simulink model "schem_3_2"  (R2024a)
settings: Solver=VariableStepAuto  StartTime=0.0  StopTime=25  RelTol=1e-3
undefined symbols (not defined in the file): G11, G12, G21, G22, G23, xi_120, xi_220, xi_230
settings Model: Creator=user  LastModifiedBy=user

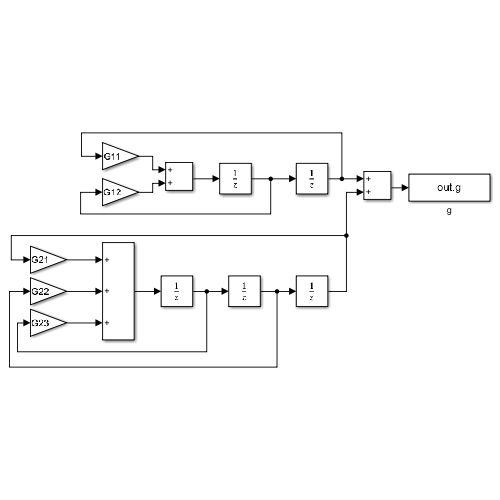
[thumbnail: Simulink's stored preview of the top-level diagram]
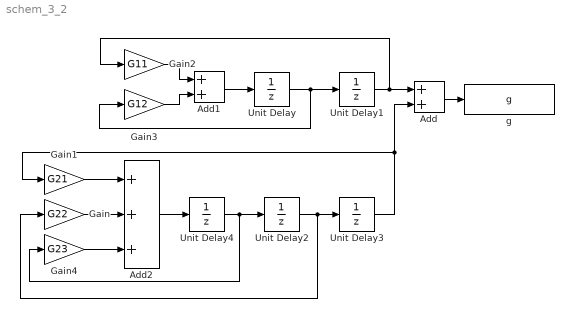
== system schem_3_2 ==
  Add : Sum
  Add1 : Sum
  Add2 : Sum  Inputs=+++
  Gain : Gain  Gain=G22
  Gain1 : Gain  Gain=G21
  Gain2 : Gain  Gain=G11
  Gain3 : Gain  Gain=G12
  Gain4 : Gain  Gain=G23
  Unit Delay : UnitDelay  InitialCondition=xi_120  SampleTime=0.25  HasFrameUpgradeWarning=on
  Unit Delay1 : UnitDelay  SampleTime=0.25  HasFrameUpgradeWarning=on
  Unit Delay2 : UnitDelay  InitialCondition=xi_220  SampleTime=0.25  HasFrameUpgradeWarning=on
  Unit Delay3 : UnitDelay  SampleTime=0.25  HasFrameUpgradeWarning=on
  Unit Delay4 : UnitDelay  InitialCondition=xi_230  SampleTime=0.25  HasFrameUpgradeWarning=on
  g : ToWorkspace  VariableName=g  SaveFormat=Timeseries  SampleTime=-1
  wires:
  Unit Delay/1 -> Gain3/1, Unit Delay1/1
  Add/1 -> g/1
  Add1/1 -> Unit Delay/1
  Gain2/1 -> Add1/1
  Gain3/1 -> Add1/2
  Unit Delay1/1 -> Gain2/1, Add/1
  Add2/1 -> Unit Delay4/1
  Gain1/1 -> Add2/1
  Unit Delay2/1 -> Gain/1, Unit Delay3/1
  Unit Delay3/1 -> Add/2, Gain1/1
  Unit Delay4/1 -> Gain4/1, Unit Delay2/1
  Gain/1 -> Add2/2
  Gain4/1 -> Add2/3
